simulink model "full_system_nios"  (R2021b)
settings: Solver=FixedStepDiscrete  StartTime=0.0  StopTime=250000  RelTol=1e-3
model workspace (MAT data in the model file):
  out_size = 0
undefined symbols (not defined in the file): betas, bias, DiscIntNeverNeededParam, mus, scale, sigmas
libraries: hdlsllib x2
(part 3 of 3)

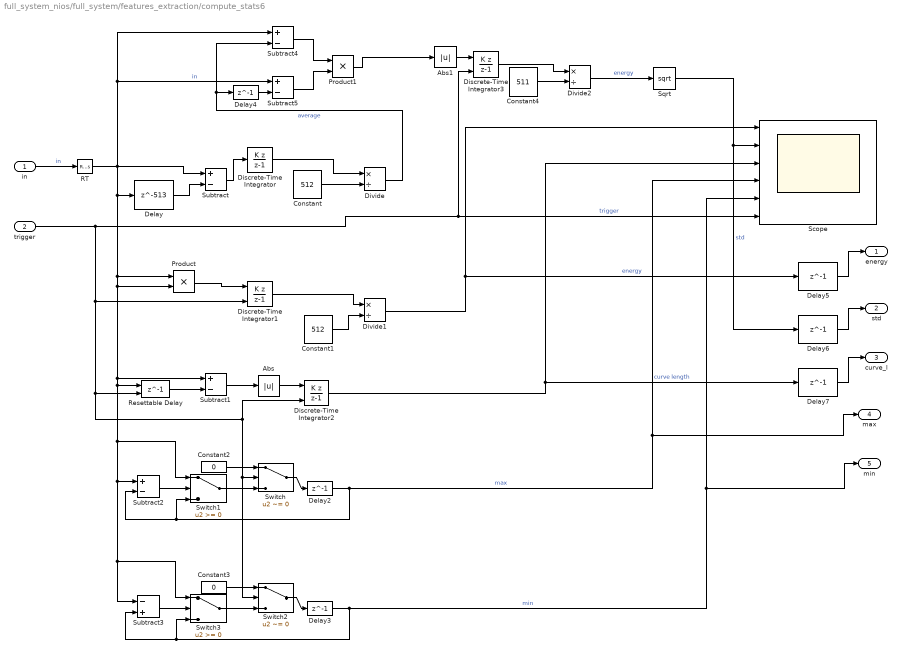
== system full_system_nios/full_system/features_extraction/compute_stats6 ==
  in : Inport
  trigger : Inport  Port=2
  Abs : Abs
  Abs1 : Abs
  Constant : Constant  Value=512  VectorParams1D=off  OutDataTypeStr=uint16  SampleTime=-1
  Constant1 : Constant  Value=512  VectorParams1D=off  OutDataTypeStr=uint16  SampleTime=-1
  Constant2 : Constant  Value=0  VectorParams1D=off  OutDataTypeStr=uint8  SampleTime=-1
  Constant3 : Constant  Value=0  VectorParams1D=off  OutDataTypeStr=uint8  SampleTime=-1
  Constant4 : Constant  Value=511  VectorParams1D=off  OutDataTypeStr=uint16  SampleTime=-1
  Delay : Delay  DelayLength=513  InitialCondition=0  UseCircularBuffer=on
  Delay{2..7} (6 alike) : Delay  DelayLength=1  InitialCondition=0  UseCircularBuffer=on
  Discrete-Time Integrator : DiscreteIntegrator  IntegratorMethod=Accumulation: Backward Euler  SampleTime=-1  ICPrevOutput=DiscIntNeverNeededParam  ICPrevScaledInput=DiscIntNeverNeededParam
  Discrete-Time Integrator1 : DiscreteIntegrator  IntegratorMethod=Accumulation: Backward Euler  ExternalReset=rising  SampleTime=-1  ICPrevOutput=DiscIntNeverNeededParam  ICPrevScaledInput=DiscIntNeverNeededParam
  Discrete-Time Integrator2 : DiscreteIntegrator  IntegratorMethod=Accumulation: Backward Euler  ExternalReset=rising  SampleTime=-1  ICPrevOutput=DiscIntNeverNeededParam  ICPrevScaledInput=DiscIntNeverNeededParam
  Discrete-Time Integrator3 : DiscreteIntegrator  IntegratorMethod=Accumulation: Backward Euler  ExternalReset=rising  SampleTime=-1  ICPrevOutput=DiscIntNeverNeededParam  ICPrevScaledInput=DiscIntNeverNeededParam
  Divide : Product  Inputs=*/  RndMeth=Zero  SaturateOnIntegerOverflow=on  OutDataTypeStr=Inherit: Same as first input
  Divide1 : Product  Inputs=*/  RndMeth=Zero  SaturateOnIntegerOverflow=on
  Divide2 : Product  Inputs=*/  RndMeth=Zero  SaturateOnIntegerOverflow=on
  Product : Product
  Product1 : Product
  RT : RateTransition  OutPortSampleTime=1
  Resettable Delay : Delay  DelayLength=1  ExternalReset=Level
      settings: InputPortMap=u0,r5
  Scope : Scope  NumInputPorts=6
  Sqrt : Sqrt  SaturateOnIntegerOverflow=on
  Subtract{,1..2,4..5} (5 alike) : Sum  Inputs=+-
  Subtract3 : Sum  Inputs=-+
  Switch : Switch  Criteria=u2 ~= 0
  Switch1 : Switch  OutDataTypeStr=Inherit: Same as first input
  Switch2 : Switch  Criteria=u2 ~= 0
  Switch3 : Switch  OutDataTypeStr=Inherit: Same as first input
  energy : Outport
  std : Outport  Port=2
  curve_l : Outport  Port=3
  max : Outport  Port=4
  min : Outport  Port=5
  wires:
  Constant/1 -> Divide/2
  Subtract/1 -> Discrete-Time Integrator/1
  Delay/1 -> Subtract/2
  Product/1 -> Discrete-Time Integrator1/1
  Constant1/1 -> Divide1/2
  Resettable Delay/1 -> Subtract1/2
  Subtract1/1 -> Abs/1
  Abs/1 -> Discrete-Time Integrator2/1
  Discrete-Time Integrator2/1 -> Delay7/1, Scope/3  "curve length"
  Constant2/1 -> Switch/1
  Subtract2/1 -> Switch1/2
  Delay2/1 -> max/1, Scope/4, Switch1/3, Subtract2/2  "max"
  Switch/1 -> Delay2/1
  Switch1/1 -> Switch/3
  Constant3/1 -> Switch2/1
  Switch2/1 -> Delay3/1
  Switch3/1 -> Switch2/3
  Subtract3/1 -> Switch3/2
  Delay3/1 -> min/1, Scope/5, Switch3/3, Subtract3/2  "min"
  trigger/1 -> Discrete-Time Integrator3/2, Scope/6, Discrete-Time Integrator1/2, Resettable Delay/2, Discrete-Time Integrator2/2, Switch2/2, Switch/2  "trigger"
  RT/1 -> Subtract4/1, Subtract5/1, Delay/1, Product/1, Switch1/1, Switch3/1, Subtract3/1, Subtract2/1, Resettable Delay/1, Subtract1/1, Product/2, Subtract/1  "in"
  Delay4/1 -> Subtract5/2
  Subtract4/1 -> Product1/1
  Subtract5/1 -> Product1/2
  Constant4/1 -> Divide2/2
  Discrete-Time Integrator3/1 -> Divide2/1
  Divide/1 -> Subtract4/2, Delay4/1  "average"
  Discrete-Time Integrator/1 -> Divide/1
  Divide2/1 -> Sqrt/1  "energy"
  Abs1/1 -> Discrete-Time Integrator3/1
  Delay5/1 -> energy/1
  Delay6/1 -> std/1
  Delay7/1 -> curve_l/1
  Divide1/1 -> Scope/1, Delay5/1  "energy"
  Sqrt/1 -> Scope/2, Delay6/1  "std"
  in/1 -> RT/1  "in"
  Product1/1 -> Abs1/1
  Discrete-Time Integrator1/1 -> Divide1/1

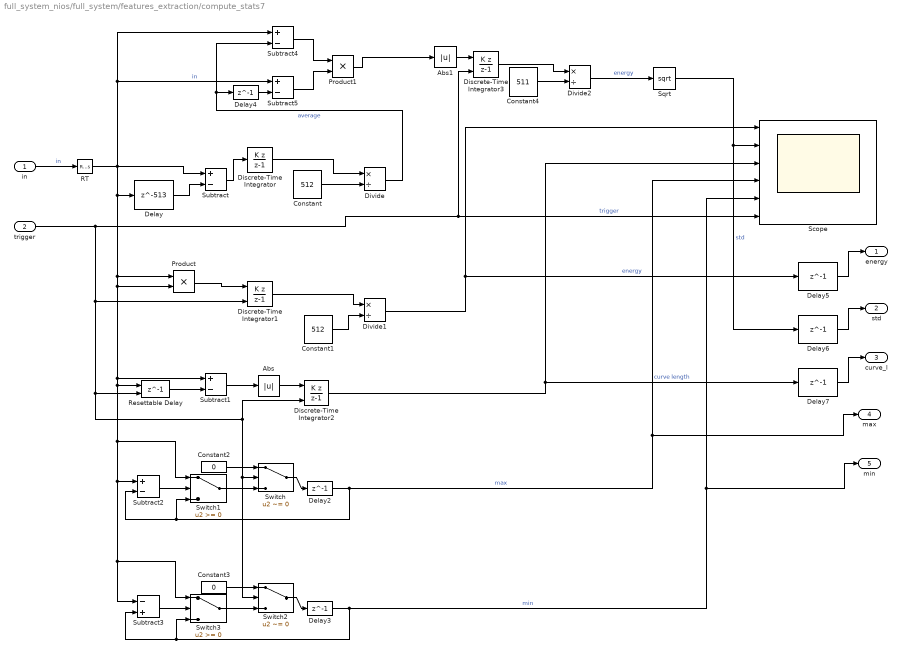
== system full_system_nios/full_system/features_extraction/compute_stats7 ==
  in : Inport
  trigger : Inport  Port=2
  Abs : Abs
  Abs1 : Abs
  Constant : Constant  Value=512  VectorParams1D=off  OutDataTypeStr=uint16  SampleTime=-1
  Constant1 : Constant  Value=512  VectorParams1D=off  OutDataTypeStr=uint16  SampleTime=-1
  Constant2 : Constant  Value=0  VectorParams1D=off  OutDataTypeStr=uint8  SampleTime=-1
  Constant3 : Constant  Value=0  VectorParams1D=off  OutDataTypeStr=uint8  SampleTime=-1
  Constant4 : Constant  Value=511  VectorParams1D=off  OutDataTypeStr=uint16  SampleTime=-1
  Delay : Delay  DelayLength=513  InitialCondition=0  UseCircularBuffer=on
  Delay{2..7} (6 alike) : Delay  DelayLength=1  InitialCondition=0  UseCircularBuffer=on
  Discrete-Time Integrator : DiscreteIntegrator  IntegratorMethod=Accumulation: Backward Euler  SampleTime=-1  ICPrevOutput=DiscIntNeverNeededParam  ICPrevScaledInput=DiscIntNeverNeededParam
  Discrete-Time Integrator1 : DiscreteIntegrator  IntegratorMethod=Accumulation: Backward Euler  ExternalReset=rising  SampleTime=-1  ICPrevOutput=DiscIntNeverNeededParam  ICPrevScaledInput=DiscIntNeverNeededParam
  Discrete-Time Integrator2 : DiscreteIntegrator  IntegratorMethod=Accumulation: Backward Euler  ExternalReset=rising  SampleTime=-1  ICPrevOutput=DiscIntNeverNeededParam  ICPrevScaledInput=DiscIntNeverNeededParam
  Discrete-Time Integrator3 : DiscreteIntegrator  IntegratorMethod=Accumulation: Backward Euler  ExternalReset=rising  SampleTime=-1  ICPrevOutput=DiscIntNeverNeededParam  ICPrevScaledInput=DiscIntNeverNeededParam
  Divide : Product  Inputs=*/  RndMeth=Zero  SaturateOnIntegerOverflow=on  OutDataTypeStr=Inherit: Same as first input
  Divide1 : Product  Inputs=*/  RndMeth=Zero  SaturateOnIntegerOverflow=on
  Divide2 : Product  Inputs=*/  RndMeth=Zero  SaturateOnIntegerOverflow=on
  Product : Product
  Product1 : Product
  RT : RateTransition  OutPortSampleTime=1
  Resettable Delay : Delay  DelayLength=1  ExternalReset=Level
      settings: InputPortMap=u0,r5
  Scope : Scope  NumInputPorts=6
  Sqrt : Sqrt  SaturateOnIntegerOverflow=on
  Subtract{,1..2,4..5} (5 alike) : Sum  Inputs=+-
  Subtract3 : Sum  Inputs=-+
  Switch : Switch  Criteria=u2 ~= 0
  Switch1 : Switch  OutDataTypeStr=Inherit: Same as first input
  Switch2 : Switch  Criteria=u2 ~= 0
  Switch3 : Switch  OutDataTypeStr=Inherit: Same as first input
  energy : Outport
  std : Outport  Port=2
  curve_l : Outport  Port=3
  max : Outport  Port=4
  min : Outport  Port=5
  wires:
  Constant/1 -> Divide/2
  Subtract/1 -> Discrete-Time Integrator/1
  Delay/1 -> Subtract/2
  Product/1 -> Discrete-Time Integrator1/1
  Constant1/1 -> Divide1/2
  Resettable Delay/1 -> Subtract1/2
  Subtract1/1 -> Abs/1
  Abs/1 -> Discrete-Time Integrator2/1
  Discrete-Time Integrator2/1 -> Delay7/1, Scope/3  "curve length"
  Constant2/1 -> Switch/1
  Subtract2/1 -> Switch1/2
  Delay2/1 -> max/1, Scope/4, Switch1/3, Subtract2/2  "max"
  Switch/1 -> Delay2/1
  Switch1/1 -> Switch/3
  Constant3/1 -> Switch2/1
  Switch2/1 -> Delay3/1
  Switch3/1 -> Switch2/3
  Subtract3/1 -> Switch3/2
  Delay3/1 -> min/1, Scope/5, Switch3/3, Subtract3/2  "min"
  trigger/1 -> Discrete-Time Integrator3/2, Scope/6, Discrete-Time Integrator1/2, Resettable Delay/2, Discrete-Time Integrator2/2, Switch2/2, Switch/2  "trigger"
  RT/1 -> Subtract4/1, Subtract5/1, Delay/1, Product/1, Switch1/1, Switch3/1, Subtract3/1, Subtract2/1, Resettable Delay/1, Subtract1/1, Product/2, Subtract/1  "in"
  Delay4/1 -> Subtract5/2
  Subtract4/1 -> Product1/1
  Subtract5/1 -> Product1/2
  Constant4/1 -> Divide2/2
  Discrete-Time Integrator3/1 -> Divide2/1
  Divide/1 -> Subtract4/2, Delay4/1  "average"
  Discrete-Time Integrator/1 -> Divide/1
  Divide2/1 -> Sqrt/1  "energy"
  Abs1/1 -> Discrete-Time Integrator3/1
  Delay5/1 -> energy/1
  Delay6/1 -> std/1
  Delay7/1 -> curve_l/1
  Divide1/1 -> Scope/1, Delay5/1  "energy"
  Sqrt/1 -> Scope/2, Delay6/1  "std"
  in/1 -> RT/1  "in"
  Product1/1 -> Abs1/1
  Discrete-Time Integrator1/1 -> Divide1/1
